simulink model "sampleModel245"  (R2021b)
settings: Solver=VariableStepAuto  StartTime=0.0  StopTime=10.0  RelTol=1e-3
undefined symbols (not defined in the file or in its folder): DiscIntNeverNeededParam
libraries: simulink x4, slpidlib x1
settings Model: Creator=user  LastModifiedBy=user

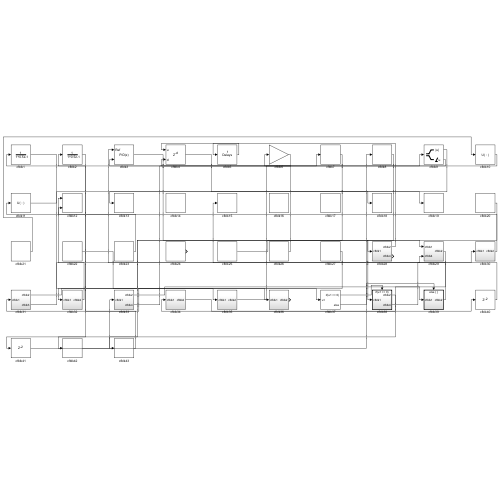
[thumbnail: Simulink's stored preview of the top-level diagram]
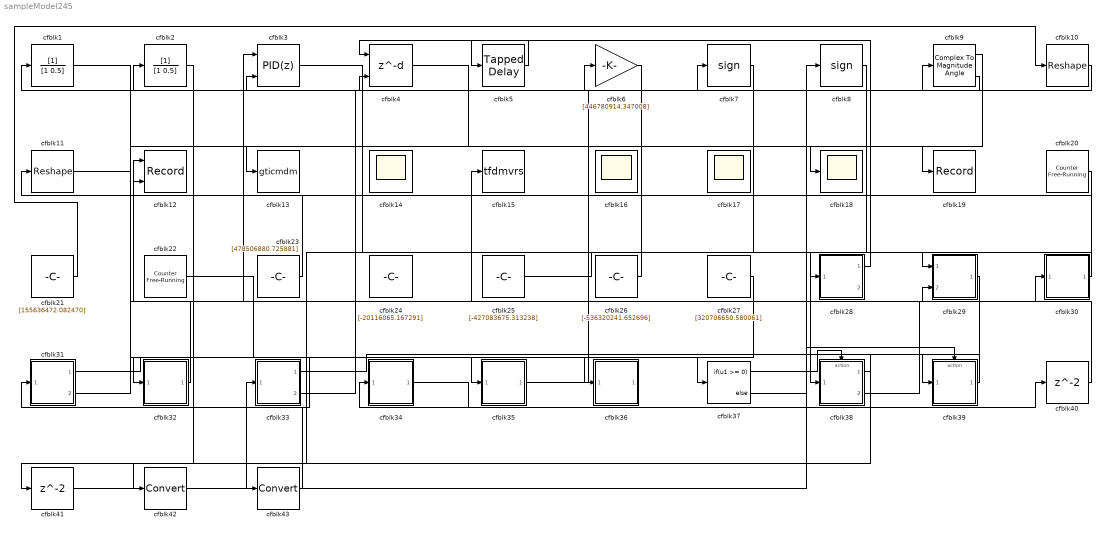
== system sampleModel245 ==
  cfblk1 : DiscreteFilter  SampleTime=1
  cfblk10 : Reshape
  cfblk11 : Reshape
  cfblk12 : Record  FileSettingsInternal="{\"entries\":[{\"content\":{\"excelSettings\":{\"content\":{},\"type\":\"Streamout.ExcelSettings\"}},\"type\":\"Streamout.FileSettingStorage\",\"uuid\":\"a42234f3-ce43-4d62-8183-94350aca9a07\"}],\"packageUris\":[\"http://schema.mathworks.com/mf0/streamout_blocks/R2020a\"],\"version\":\"1.0\"}"  Layout=[1 1]  SignalsInternal="{\"entries\":[{\"content\":{\"signals\":[{\"content\":{\"blockPath\":[\"sampleModel245/cfblk12\"],\"channel\":[],\"dimensions\":[1],\"domain\":\"sampleModel245/cfblk12\",\"lineColor\":\"#a2142f\",\"plots\":[1],\"port\":1,\"sid\":[\"\"],\"signalID\":9842,\"signalName\":\"cfblk32\"},\"type\":\"RecordBlkView.Signal\",\"uuid\":\"6b7f1dfd-fd8e-4140-a1dc-e27f85fc05a0\"},{\"content\":{\"blockPath\":[\"sampleModel245/cfblk12\"],\"channel\":[],\"dimensions\":[1],\"domain\":\"sampleModel245/cfblk12\",\"lineColor\":\"#139fff\",\"plots\":[1],\"port\":2,\"sid\":[\"\"],\"signalID\":9846,\"signalName\":\"cfblk30\"},\"type\":\"RecordBlkView.Signal\",\"uuid\":\"dc324ef5-c37b-4610-8a1b-5c676834dfe0\"}]},\"type\":\"RecordBlkView.InputSignals\",\"uuid\":\"7a7d1915-d8fc-400e-b9f0-b1be9a6be0f6\"}],\"packageUris\":[\"http://schema.mathworks.com/mf0/streamout_blocks/R2020a\"],\"version\":\"1.0\"}"  VisualizationBindings="{\"xyplotplugin\":{\"info\":[{\"series\":[{\"bindingParametersList\":[{\"parameter\":\"X-Axis\",\"signalID\":9842,\"signalName\":\"cfblk32\"},{\"parameter\":\"Y-Axis\",\"signalID\":9846,\"signalName\":\"cfblk30\"}],\"seriesID\":42464}],\"subplotID\":1}]}}"  CompatibilityTag=XY
  cfblk13 : ToWorkspace  VariableName=gticmdm  SaveFormat=Timeseries  SampleTime=-1
  cfblk{14,16..18} (4 alike) : Scope
      cfblk14 settings: Floating=on
      cfblk16 settings: Floating=on
      cfblk17 settings: Floating=on
  cfblk15 : ToWorkspace  VariableName=tfdmvrs  SaveFormat=Timeseries  SampleTime=-1
  cfblk19 : Record  FileSettingsInternal="{\"entries\":[{\"content\":{\"excelSettings\":{\"content\":{},\"type\":\"Streamout.ExcelSettings\"}},\"type\":\"Streamout.FileSettingStorage\",\"uuid\":\"8d9c6872-5cdd-4d69-9216-271c63a9f369\"}],\"packageUris\":[\"http://schema.mathworks.com/mf0/streamout_blocks/R2020a\"],\"version\":\"1.0\"}"  SignalsInternal="{\"entries\":[{\"content\":{\"signals\":[{\"content\":{\"blockPath\":[\"sampleModel245/cfblk19\"],\"channel\":[],\"dimensions\":[1],\"domain\":\"sampleModel245/cfblk19\",\"lineColor\":\"#77ac30\",\"plots\":[1],\"port\":1,\"sid\":[\"\"],\"signalID\":9850,\"signalName\":\"cfblk4\"},\"type\":\"RecordBlkView.Signal\",\"uuid\":\"eaa34cd2-6ae7-4d4b-bce4-618d9346050c\"}]},\"type\":\"RecordBlkView.InputSignals\",\"uuid\":\"4a90d364-c465-433d-9f25-5f9737d349f5\"}],\"packageUris\":[\"http://schema.mathworks.com/mf0/streamout_blocks/R2020a\"],\"version\":\"1.0\"}"  VisualizationBindings="{\"sparklinesplugin\":{\"info\":[{\"bindingParametersList\":[],\"subplotID\":1}]}}"
  cfblk2 : DiscreteFilter  SampleTime=1
  cfblk20 : simulink/Sources/Counter Free-Running  NumBits=[18.000000]  tsamp=-1
  cfblk21 : Constant  Value=[155636472.082470]  SampleTime=1
  cfblk22 : simulink/Sources/Counter Free-Running  NumBits=[1.000000]  tsamp=-1
  cfblk23 : Constant  Value=[478506880.725881]  SampleTime=1
  cfblk24 : Constant  Value=[-20116065.167291]  SampleTime=1
  cfblk25 : Constant  Value=[-427083675.313238]  SampleTime=1
  cfblk26 : Constant  Value=[-536320241.652696]  SampleTime=1
  cfblk27 : Constant  Value=[320706650.580061]  SampleTime=1
  cfblk28 : Subsystem
  cfblk29 : Subsystem
  cfblk3 : slpidlib/PID Controller (2DOF)  Controller=PID  Form=Parallel  TimeDomain=Discrete-time  UseExternalTs=off  SampleTime=1  IntegratorMethod=Forward Euler  FilterMethod=Forward Euler  ControllerParametersSource=internal  P=1  I=1  D=0  UseFilter=on  N=100  b=1  c=1  TunerSelectOption=Transfer Function Based (PID Tuner App)  InitialConditionSource=internal  InitialConditionForIntegrator=0  InitialConditionForFilter=0  DifferentiatorICPrevScaledInput=0  ExternalReset=none  TrackingMode=off  Kt=1  LimitOutput=off  SatLimitsSource=internal  UpperSaturationLimit=inf  LowerSaturationLimit=-inf  LinearizeAsGain=off  AntiWindupMode=none  Kb=1  POutMin=[]  POutMax=[]  IOutMin=[]  IOutMax=[]  DOutMin=[]  DOutMax=[]  NOutMin=[]  NOutMax=[]  bOutMin=[]  bOutMax=[]  cOutMin=[]  cOutMax=[]  SumOutMin=[]  SumOutMax=[]  SaturationOutMin=[]  SaturationOutMax=[]  PParamMin=[]  PParamMax=[]  IParamMin=[]  IParamMax=[]  DParamMin=[]  DParamMax=[]  NParamMin=[]  NParamMax=[]  bParamMin=[]  bParamMax=[]  cParamMin=[]  cParamMax=[]  KbParamMin=[]  KbParamMax=[]  KtParamMin=[]  KtParamMax=[]  KbOutMin=[]  KbOutMax=[]  KtOutMin=[]  KtOutMax=[]  IntegratorOutMin=[]  IntegratorOutMax=[]  FilterOutMin=[]  FilterOutMax=[]  SumI1OutMin=[]  SumI1OutMax=[]  SumI2OutMin=[]  SumI2OutMax=[]  SumI3OutMin=[]  SumI3OutMax=[]  SumI4OutMin=[]  SumI4OutMax=[]  SumDOutMin=[]  SumDOutMax=[]  Sum1OutMin=[]  Sum1OutMax=[]  Sum2OutMin=[]  Sum2OutMax=[]  Sum3OutMin=[]  Sum3OutMax=[]  DifferentiatorOutMin=[]  DifferentiatorOutMax=[]  FilterDiffOutCoefMin=[]  FilterDiffOutCoefMax=[]  ReciprocalOutMin=[]  ReciprocalOutMax=[]  SumDenOutMin=[]  SumDenOutMax=[]  SumNumOutMin=[]  SumNumOutMax=[]  DivideOutMin=[]  DivideOutMax=[]  UdiffTsProdOutMin=[]  UdiffTsProdOutMax=[]  NTsProdOutMin=[]  NTsProdOutMax=[]  UintegralTsProdOutMin=[]  UintegralTsProdOutMax=[]  UngainTsProdOutMin=[]  UngainTsProdOutMax=[]  IntegratorContinuousStateAttributes=''  IntegratorStateMustResolveToSignalObject=off  IntegratorRTWStateStorageClass=Auto  FilterContinuousStateAttributes=''  FilterStateMustResolveToSignalObject=off  FilterRTWStateStorageClass=Auto  ParallelPVariant=InternalParameters  IdealPVariant=Disabled  IVariant=InternalParameters  DVariant=InternalParameters  bVariant=InternalParameters  cVariant=InternalParameters  IntegratorVariant=Discrete  SatVariant=Disabled  AWVariant=Passthrough  PCopyVariant=Disabled  TRVariant=Disabled  FdbkBlocksVariant=Forward  IdealPFdbkVariant=Disabled  SatFdbkVariant=Disabled  DerivativeFilterVariant=ForwardEulerFilter  NVariant=InternalParameters  NCopyVariant=Disabled  FilterICVariant=InternalICsFilter  IntegratorICVariant=InternalICs  ExternalResetVariant=Disabled  TRSumVariant=Passthrough  SumFdbkVariant=Disabled  SumVariant=Sum_PID  TsampFilterVariant=InternalTs  TsampNgainVariant=Passthrough  TsampIntegralVariant=Passthrough  ExternalSaturationOutDataTypeStr=Inherit: Same as second input
      settings: SourceProductBaseCode=SL
  cfblk30 : Subsystem
  cfblk31 : Subsystem
  cfblk32 : Subsystem
  cfblk33 : Subsystem
  cfblk34 : Subsystem
  cfblk35 : Subsystem
  cfblk36 : Subsystem
  cfblk37 : If  IfExpression=u1 >= 0  SampleTime=1
  cfblk38 : Subsystem  TreatAsAtomicUnit=on
  cfblk39 : Subsystem  TreatAsAtomicUnit=on
  cfblk4 : Delay  DelayLengthSource=Input port  SampleTime=1
      settings: InputPortMap=u0,p1
  cfblk40 : Delay  SampleTime=1
  cfblk41 : Delay  SampleTime=1
  cfblk42 : DataTypeConversion
  cfblk43 : DataTypeConversion
  cfblk5 : simulink/Discrete/Tapped Delay  vinit=0.0  samptime=-1  NumDelays=1  DelayOrder=Oldest  includeCurrent=off
  cfblk6 : Gain  Gain=[446780914.347008]
  cfblk7 : Signum
  cfblk8 : Signum
  cfblk9 : ComplexToMagnitudeAngle
  wires:
  cfblk8/1 -> cfblk38/1(cfblk1)
  cfblk23/1 -> cfblk11/1
  cfblk7/1 -> cfblk32/1(cfblk1)
  cfblk29/1(cfblk2) -> cfblk34/1(cfblk1)
  cfblk27/1 -> cfblk31/1(cfblk1)
  cfblk28/1(cfblk2) -> cfblk5/1
  cfblk33/1(cfblk2) -> cfblk39/1(cfblk1)
  cfblk33/2(cfblk4) -> cfblk9/1
  cfblk4/1 -> cfblk19/1
  cfblk35/1(cfblk2) -> cfblk7/1
  cfblk32/1(cfblk2) -> cfblk12/1
  cfblk1/1 -> cfblk35/1(cfblk1)
  cfblk31/1(cfblk2) -> cfblk37/1
  cfblk9/1 -> cfblk13/1
  cfblk25/1 -> cfblk28/1(cfblk1)
  cfblk30/1(cfblk2) -> cfblk12/2
  cfblk26/1 -> cfblk6/1
  cfblk11/1 -> cfblk18/1
  cfblk21/1 -> cfblk10/1
  cfblk38/2(cfblk4) -> cfblk30/1(cfblk1)
  cfblk9/2 -> cfblk1/1
  cfblk6/1 -> cfblk3/2
  cfblk22/1 -> cfblk36/1(cfblk1)
  cfblk3/1 -> cfblk29/1(cfblk1)
  cfblk39/1(cfblk2) -> cfblk15/1
  cfblk31/2(cfblk3) -> cfblk29/2(cfblk4)
  cfblk5/1 -> cfblk4/1
  cfblk10/1 -> cfblk4/2
  cfblk37/1 -> cfblk38/Action
  cfblk37/2 -> cfblk39/Action
  cfblk34/1(cfblk2) -> cfblk40/1
  cfblk40/1 -> cfblk3/1
  cfblk38/1(cfblk2) -> cfblk41/1
  cfblk41/1 -> cfblk8/1
  cfblk2/1 -> cfblk42/1
  cfblk42/1 -> cfblk33/1(cfblk1)
  cfblk20/1 -> cfblk43/1
  cfblk43/1 -> cfblk2/1

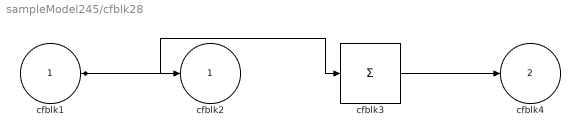
== system sampleModel245/cfblk28 ==
  cfblk1 : Inport
  cfblk3 : Sum  Inputs=+
  cfblk2 : Outport
  cfblk4 : Outport  Port=2
  wires:
  cfblk1/1 -> cfblk2/1, cfblk3/1
  cfblk3/1 -> cfblk4/1

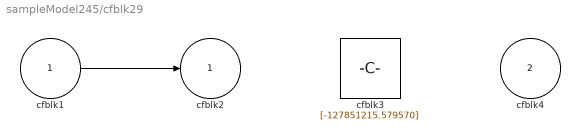
== system sampleModel245/cfblk29 ==
  cfblk1 : Inport
  cfblk4 : Inport  Port=2
  cfblk3 : Constant  Value=[-127851215.579570]  SampleTime=1
  cfblk2 : Outport
  wires:
  cfblk1/1 -> cfblk2/1

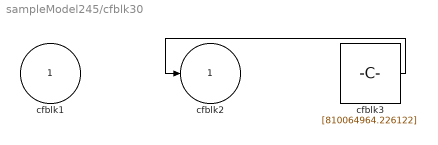
== system sampleModel245/cfblk30 ==
  cfblk1 : Inport
  cfblk3 : Constant  Value=[810064964.226122]  SampleTime=1
  cfblk2 : Outport
  wires:
  cfblk3/1 -> cfblk2/1

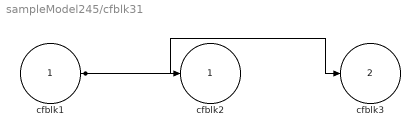
== system sampleModel245/cfblk31 ==
  cfblk1 : Inport
  cfblk2 : Outport
  cfblk3 : Outport  Port=2
  wires:
  cfblk1/1 -> cfblk3/1, cfblk2/1

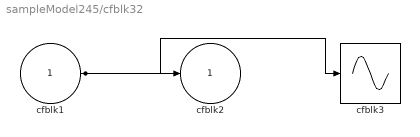
== system sampleModel245/cfblk32 ==
  cfblk1 : Inport
  cfblk3 : Sin  TimeSource=Use external signal  SampleTime=0
  cfblk2 : Outport
  wires:
  cfblk1/1 -> cfblk2/1, cfblk3/1

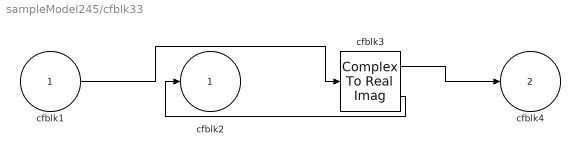
== system sampleModel245/cfblk33 ==
  cfblk1 : Inport
  cfblk3 : ComplexToRealImag
  cfblk2 : Outport
  cfblk4 : Outport  Port=2
  wires:
  cfblk3/1 -> cfblk4/1
  cfblk3/2 -> cfblk2/1
  cfblk1/1 -> cfblk3/1

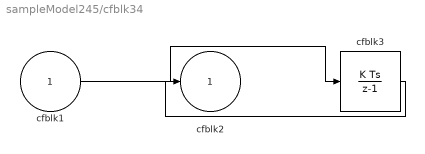
== system sampleModel245/cfblk34 ==
  cfblk1 : Inport
  cfblk3 : DiscreteIntegrator  ICPrevOutput=DiscIntNeverNeededParam  ICPrevScaledInput=DiscIntNeverNeededParam
  cfblk2 : Outport
  wires:
  cfblk1/1 -> cfblk3/1
  cfblk3/1 -> cfblk2/1

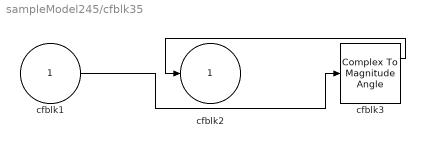
== system sampleModel245/cfblk35 ==
  cfblk1 : Inport
  cfblk3 : ComplexToMagnitudeAngle
  cfblk2 : Outport
  wires:
  cfblk3/1 -> cfblk2/1
  cfblk1/1 -> cfblk3/1

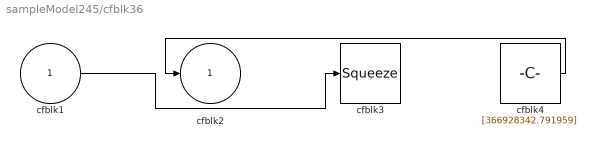
== system sampleModel245/cfblk36 ==
  cfblk1 : Inport
  cfblk3 : Squeeze
  cfblk4 : Constant  Value=[366928342.791959]  SampleTime=1
  cfblk2 : Outport
  wires:
  cfblk4/1 -> cfblk2/1
  cfblk1/1 -> cfblk3/1

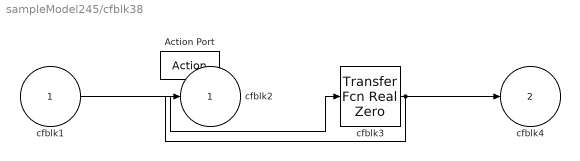
== system sampleModel245/cfblk38 ==
  cfblk1 : Inport
  Action Port : ActionPort  ActionPortLabel=if(u1 >= 0)
  cfblk3 : simulink/Discrete/Transfer Fcn Real Zero  ZeroZ=0.75  ICPrevInput=0.0  DoSatur=off
      settings: SourceProductBaseCode=SL
  cfblk2 : Outport
  cfblk4 : Outport  Port=2
  wires:
  cfblk1/1 -> cfblk3/1
  cfblk3/1 -> cfblk2/1, cfblk4/1

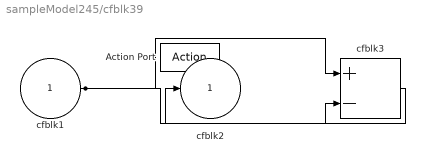
== system sampleModel245/cfblk39 ==
  cfblk1 : Inport
  Action Port : ActionPort  ActionPortLabel=else
  cfblk3 : Sum  Inputs=+-
  cfblk2 : Outport
  wires:
  cfblk3/1 -> cfblk2/1
  cfblk1/1 -> cfblk3/1, cfblk3/2
